simulink model "FOC_Motor_Sensorless"  (R2025b)
settings: Solver=VariableStepAuto  StartTime=0.0  StopTime=8  RelTol=1e-3
undefined symbols (not defined in the file or in its folder): adc, dataRange, encoder, inverter, paramAdcAmperePerCount, paramAdcCalibrationSamples, paramAdcCountAtZeroAmpere, paramAdcEnablecalibration, paramCurrentControlSatVoltage, paramOverCurrentDuration, paramOverCurrentEnable, paramOverCurrentLimit, paramPwmCompareAtZeroVolt, paramPwmCompareMax, paramPwmComparePerVolt, paramVelocityControlSatCurrent, PI_params, pmsm, PU_System, pwm, sampleTime
libraries: fl_lib x12, nesl_utility x12, mcbeeMathTransformLib x5, mcbcontrolslib x5, ee_lib x4, slpidlib x2, simulink x2, mcbhdlpositiondecoderlib x2, mcbplantlib x1, autolibpmsmexterior x1, eeGeneralControl x1, SignalEditorBlockLib x1
(part 1 of 2)
settings Model: DataDictionary=FoCFpgaData.sldd  ExtModeTrigDuration=100  LastModifiedBy=Admin
settings SolverCC: ZeroCrossAlgorithm=Adaptive  AlgebraicLoopSolver=TrustRegion
settings DataIOCC: LimitDataPoints=on  SaveFormat=Structure  SaveOutput=off  InspectSignalLogs=on  SaveTime=off  ReturnWorkspaceOutputs=off
settings OptimizationCC: DefaultParameterBehavior=Inlined  UseDivisionForNetSlopeComputation=on  GainParamInheritBuiltInType=on  UseFloatMulNetSlope=on  DefaultUnderspecifiedDataType=single  UseSpecifiedMinMax=on  InlineInvariantSignals=on  ReuseModelBlockBuffer=off  PassReuseOutputArgsAs=Individual arguments  ZeroExternalMemoryAtStartup=off  ZeroInternalMemoryAtStartup=off  NoFixptDivByZeroProtection=on  EfficientFloat2IntCast=on  LifeSpan=1  MaxStackSize=64  OptimizationLevel=level1  OptimizationCustomize=off  EfficientTunableParamExpr=on
settings DebuggingCC: IgnoredZcDiagnostic=none  SolverPrmCheckMsg=warning  InheritedTsInSrcMsg=none  ParameterPrecisionLossMsg=none  UnconnectedInputMsg=warning  UnconnectedOutputMsg=warning  UnconnectedLineMsg=warning  AllowSymbolicDim=off  SubsystemReferenceDiagnosticForUnitTest=warning  SFUnexpectedBacktrackingDiag=warning  SFNoUnconditionalDefaultTransitionDiag=warning  SFExecutionAtInitializationDiag=none  ArithmeticOperatorsInVariantConditions=warning
settings HardwareCC: ProdBitPerPointer=32.0  ProdBitPerSizeT=32.0  ProdBitPerPtrDiffT=32.0  ProdLargestAtomicInteger=Long  ProdWordSize=32.0  ProdLongLongMode=on  ProdHWDeviceType=ARM Compatible->ARM 10  TargetBitPerPointer=64.0  TargetBitPerSizeT=64.0  TargetBitPerPtrDiffT=64.0  TargetLongLongMode=on  TargetIntDivRoundTo=Zero  TargetEndianess=LittleEndian  TargetWordSize=64.0  TargetHWDeviceType=MATLAB Host  ProdEqTarget=off
settings ModelReferenceCC: EnableRefExpFcnMdlSchedulingChecks=on  PropagateSignalLabelsOutOfModel=off
settings SFSimCC: SimUseLocalCustomCode=off  MATLABDynamicMemAlloc=off  CustomCodeUndefinedFunction=UseInterfaceOnly
settings RTWCC: SystemTargetFile=ert.tlc  TemplateMakefile=ert_default_tmf  GenerateReport=on  RTWUseLocalCustomCode=off  BuildConfiguration=Faster Runs  IncludeHyperlinkInReport=on  LaunchReport=on  CodeProfilingSaveOptions=AllData  DataTypeReplacement=CDataTypesFixedWidth  TargetLang=C++  GenerateTraceInfo=on  GenerateCodeMetricsReport=on  GPUComputeCapability=3.5  DLArmComputeVersion=19.05  Description=Embedded Coder
settings CodeAppCC: ForceParamTrailComments=on  GenerateComments=off  IgnoreCustomStorageClasses=off  SimulinkDataObjDesc=on  CustomSymbolStrGlobalVar=rt$N$M  CustomSymbolStrType=$N$M  CustomSymbolStrFcn=$N$M$F  CustomSymbolStrFcnArg=$I$N$M  CustomSymbolStrMacro=$N$M  InsertBlockDesc=on
settings ERTTargetCC: RootIOFormat=Structure reference  ERTCustomFileTemplate=example_file_process.tlc  ERTFilePackagingFormat=CompactWithDataFile  PreserveExternInFcnDecls=off  EnableSignedLeftShifts=off  EnableSignedRightShifts=off  MaxIdInt64=INT64_MAX  MinIdInt64=INT64_MIN  MaxIdUint64=UINT64_MAX  MaxIdInt32=INT32_MAX  MinIdInt32=INT32_MIN  MaxIdUint32=UINT32_MAX  MaxIdInt16=INT16_MAX  MinIdInt16=INT16_MIN  MaxIdUint16=UINT16_MAX  MaxIdInt8=INT8_MAX  MinIdInt8=INT8_MIN  MaxIdUint8=UINT8_MAX  TargetLangStandard=C++17 (ISO)  MultiwordLength=2048.0  GenerateSampleERTMain=on  IncludeMdlTerminateFcn=off  CombineSignalStateStructs=on  CodeInterfacePackaging=C++ class  SubcomponentCodeInterfacePackaging=C++ class  SupportComplex=off  SupportNonInlinedSFcns=on
settings ConfigComp: CovMetricSettings=dw  CovSaveCumulativeToWorkspaceVar=on  CovSaveSingleToWorkspaceVar=on  CovExternalEMLEnable=off  CovSFcnEnable=off  PLC_TargetIDE=codesys35  PLC_MultiTBSigbuilderTimeRange=off  PLC_FoldFBCallOutputVar=off  PLC_RemoveUnusedSSMethodCallArguments=off  PLC_UseCallOutputArgSyntax=off  PLC_EnableUnsignedAndDoubleTypes=off  PLC_EnableUDTSplitting=off  PLC_MaxFieldsInUDT=500.0  PLC_InlineEnumCastFunction=off  PLC_RTWMaxIdLength=31.0  PLC_RollThreshold=5.0  PLC_ActiveTab=0.0  PLC_EnableStringLiteralTB=on  PLC_Enable64bitIntSupport=off
settings SimscapeCC: SimscapeNormalizeSystem=off  SimscapeNominalValues="[{\"value\":\"10\",\"unit\":\"V\"},{\"value\":\"1\",\"unit\":\"A\"},{\"value\":\"10\",\"unit\":\"N*m\"},{\"value\":\"10\",\"unit\":\"bar\"},{\"value\":\"100\",\"unit\":\"kJ/kg\"},{\"value\":\"1\",\"unit\":\"kW\"},{\"value\":\"300\",\"unit\":\"K\"},{\"value\":\"100\",\"unit\":\"cm^3/s\"},{\"value\":\"1\",\"unit\":\"kN\"},{\"value\":\"1\",\"unit\":\"g/cm^3\"},{\"value\":\"1\",\"unit\":\"l\"},{\"value\":\"1\",\"unit\":\"cm^2\"},{\"value\":\"60\",\"unit\":\"Hz\"}]"
settings SettingsController: CoderTargetData=[]

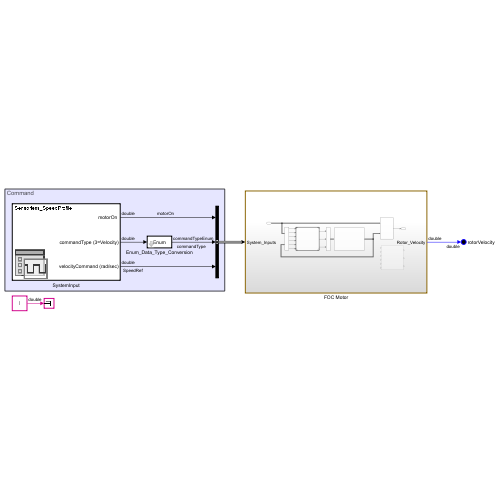
[thumbnail: Simulink's stored preview of the top-level diagram]
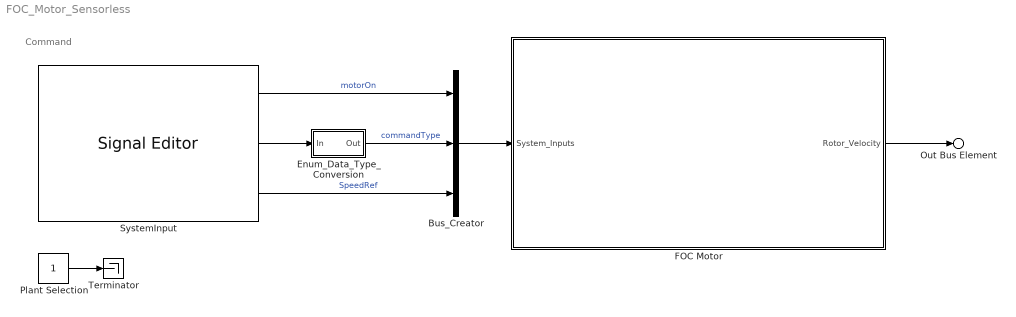
== system FOC_Motor_Sensorless ==
  note: Command
  Bus_Creator : BusCreator  Inputs=3
  Enum_Data_Type_Conversion : Subsystem  mask(Convert to enumerated data type){dataTypeStr=Enum: commandTypeEnum}
      mask prompts: dataTypeStr "Output data type"
      mask Display: disp('Enum')
  FOC Motor : Subsystem
  Plant Selection : Constant
  SystemInput : SignalEditorBlockLib/Signal Editor  FileName=SystemInputFO.mat  ActiveScenario=Sensorless_SpeedProfile  ActiveSignal=motorOn  IsBus=off  OutputBusObjectStr=Bus: BusObject  SampleTime=0  Interpolate=off  ZeroCross=off  OutputAfterFinalValue=Setting to zero  Unit=inherit  PreserveSignalName=on  ApplySigPropsToAllScenarios=off  ApplySigPropsToAllSignals=off  SignalPropertySource=Dialog parameters
  Terminator : Terminator
  Out Bus Element : Outport  PortName=rotorVelocity
  wires:
  Plant Selection/1 -> Terminator/1
  FOC Motor/1(Rotor_Velocity) -> Out Bus Element/1
  Bus_Creator/1 -> FOC Motor/1(System_Inputs)
  SystemInput/3 -> Bus_Creator/3  "SpeedRef"
  Enum_Data_Type_Conversion/1(Out) -> Bus_Creator/2  "commandType"
  SystemInput/2 -> Enum_Data_Type_Conversion/1(In)
  SystemInput/1 -> Bus_Creator/1  "motorOn"

== system FOC_Motor_Sensorless/Enum_Data_Type_Conversion ==
  note: Enum Data Type Conversion
  In : Inport
  Enum_Data_Type : DataTypeConversion  OutDataTypeStr=Enum: commandTypeEnum  SaturateOnIntegerOverflow=off  RndMeth=Floor
  Int32_Data_Type : DataTypeConversion  OutDataTypeStr=int32  SaturateOnIntegerOverflow=off  RndMeth=Floor
  Out : Outport
  wires:
  In/1 -> Int32_Data_Type/1
  Int32_Data_Type/1 -> Enum_Data_Type/1
  Enum_Data_Type/1 -> Out/1

== system FOC_Motor_Sensorless/FOC Motor ==
  note: Permanent Magnet Synchronous Motor Field Oriented Control
  System_Inputs : Inport
  Continuous_To_Discrete : Subsystem
      mask Display: fprintf('C/D')
  Controller_Algorithm_Local : Subsystem  Commented=on  TreatAsAtomicUnit=on  DataTypeOverrideAppliesTo=Fixed-point
      mask Display: image('MC_Mask.jpg');
  Discrete_To_Continuous : Subsystem  Description=""
      mask Display: fprintf('D/C')
  Model : ModelReference  ModelNameDialog=Controller_Algorithm_Local_FO.slx  SimulationMode=Normal  ModelReferenceVersion=1.4
  Motor_And_Load : Subsystem
      mask Display: image('mcb_pmsmfoc_motor.png');
  Verify_Outputs : Subsystem  Description=|
      | System Analysis for Speed Control Design
      | 
      | Analyize and plot signals used to analyize performance of
      | speed  control designs
      mask Display: fprintf('Verify\nOutputs')
  Rotor_Velocity : Outport
  wires:
  Continuous_To_Discrete/5(Encoder_Index_Found) -> Model/5
  Continuous_To_Discrete/4(ADC_Count) -> Model/4
  Motor_And_Load/1(Out) -> Continuous_To_Discrete/2(Motor_Measurements), Verify_Outputs/2(System_Measurements)
  Model/1 -> Discrete_To_Continuous/1(Controller_Mode)
  Discrete_To_Continuous/1(Motor_Commands) -> Motor_And_Load/1(Controller)
  Model/3 -> Discrete_To_Continuous/3(PWM_Compare)
  Continuous_To_Discrete/1(Motor_On) -> Model/1
  System_Inputs/1 -> Continuous_To_Discrete/1(System_Inputs), Verify_Outputs/1(System_Inputs)
  Continuous_To_Discrete/3(Velocity_Command) -> Model/3
  Verify_Outputs/1(Rotor_Velocity) -> Rotor_Velocity/1
  Continuous_To_Discrete/2(Command_Type) -> Model/2
  Continuous_To_Discrete/6(Encoder_Count) -> Model/6
  Model/2 -> Discrete_To_Continuous/2(Inverter_Enable)

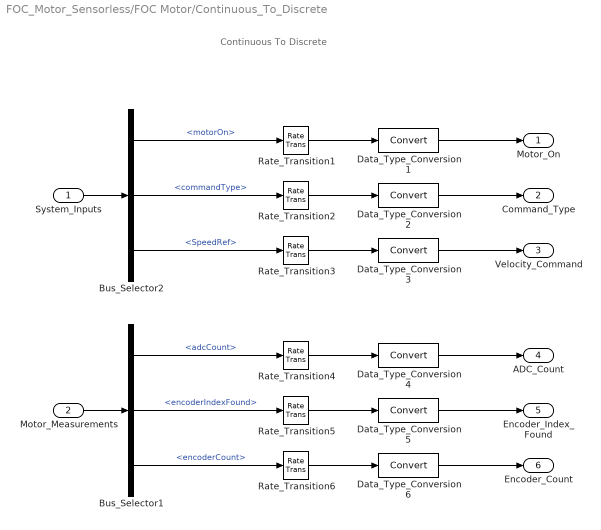
== system FOC_Motor_Sensorless/FOC Motor/Continuous_To_Discrete ==
  note: Continuous To Discrete
  System_Inputs : Inport
  Motor_Measurements : Inport  Port=2
  Bus_Selector1 : BusSelector  OutputSignals=adcCount,encoderIndexFound,encoderCount
  Bus_Selector2 : BusSelector  OutputSignals=motorOn,commandType,SpeedRef
  Data_Type_Conversion{1..6} (6 alike) : DataTypeConversion  SaturateOnIntegerOverflow=off  RndMeth=Floor
  Rate_Transition1 : RateTransition  Integrity=off  Deterministic=off
  Rate_Transition2 : RateTransition  Integrity=off  Deterministic=off
  Rate_Transition3 : RateTransition  Integrity=off  Deterministic=off
  Rate_Transition4 : RateTransition  Deterministic=off
  Rate_Transition5 : RateTransition  Deterministic=off
  Rate_Transition6 : RateTransition  Deterministic=off
  Motor_On : Outport
  Command_Type : Outport  Port=2
  Velocity_Command : Outport  Port=3
  ADC_Count : Outport  Port=4
  Encoder_Index_Found : Outport  Port=5
  Encoder_Count : Outport  Port=6
  wires:
  Bus_Selector2/3 -> Rate_Transition3/1  "<SpeedRef>"
  Bus_Selector2/2 -> Rate_Transition2/1  "<commandType>"
  Bus_Selector2/1 -> Rate_Transition1/1  "<motorOn>"
  System_Inputs/1 -> Bus_Selector2/1
  Bus_Selector1/3 -> Rate_Transition6/1  "<encoderCount>"
  Bus_Selector1/2 -> Rate_Transition5/1  "<encoderIndexFound>"
  Bus_Selector1/1 -> Rate_Transition4/1  "<adcCount>"
  Data_Type_Conversion6/1 -> Encoder_Count/1
  Data_Type_Conversion5/1 -> Encoder_Index_Found/1
  Rate_Transition6/1 -> Data_Type_Conversion6/1
  Rate_Transition5/1 -> Data_Type_Conversion5/1
  Rate_Transition1/1 -> Data_Type_Conversion1/1
  Data_Type_Conversion1/1 -> Motor_On/1
  Motor_Measurements/1 -> Bus_Selector1/1
  Data_Type_Conversion4/1 -> ADC_Count/1
  Rate_Transition4/1 -> Data_Type_Conversion4/1
  Rate_Transition3/1 -> Data_Type_Conversion3/1
  Data_Type_Conversion3/1 -> Velocity_Command/1
  Data_Type_Conversion2/1 -> Command_Type/1
  Rate_Transition2/1 -> Data_Type_Conversion2/1

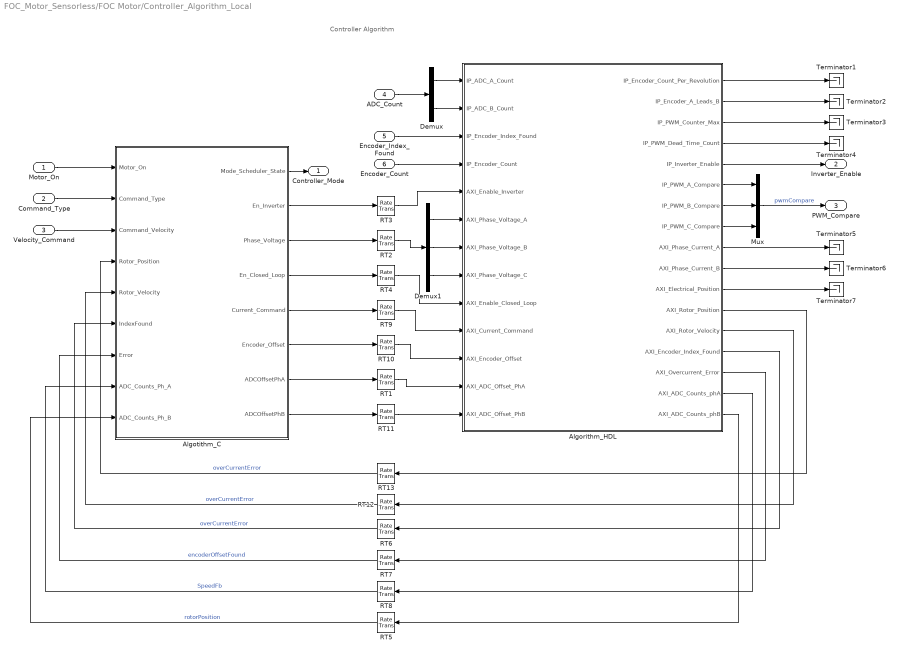
== system FOC_Motor_Sensorless/FOC Motor/Controller_Algorithm_Local ==
  note: Controller Algorithm
  Motor_On : Inport  SampleTime=sampleTime.VelocityControl  Interpolate=off
  Command_Type : Inport  Port=2  Interpolate=off
  Velocity_Command : Inport  Port=3
  ADC_Count : Inport  Port=4  PortDimensions=2  SampleTime=sampleTime.CurrentControl  Interpolate=off
  Encoder_Index_Found : Inport  Port=5  Interpolate=off
  Encoder_Count : Inport  Port=6  Interpolate=off
  Algorithm_HDL : Subsystem
  Algotithm_C : Subsystem
  Demux : Demux  Outputs=2
  Demux1 : Demux  Outputs=3
  Mux : Mux  Inputs=3
  RT{1..13} (13 alike) : RateTransition  Integrity=off
  Terminator{1..7} (7 alike) : Terminator
  Controller_Mode : Outport
  Inverter_Enable : Outport  Port=2
  PWM_Compare : Outport  Port=3
  wires:
  ADC_Count/1 -> Demux/1
  Mux/1 -> PWM_Compare/1  "pwmCompare"
  RT2/1 -> Demux1/1
  Motor_On/1 -> Algotithm_C/1(Motor_On)
  Command_Type/1 -> Algotithm_C/2(Command_Type)
  Velocity_Command/1 -> Algotithm_C/3(Command_Velocity)
  RT13/1 -> Algotithm_C/4(Rotor_Position)  "overCurrentError"
  RT12/1 -> Algotithm_C/5(Rotor_Velocity)  "overCurrentError"
  RT6/1 -> Algotithm_C/6(IndexFound)  "overCurrentError"
  RT7/1 -> Algotithm_C/7(Error)  "encoderOffsetFound"
  RT8/1 -> Algotithm_C/8(ADC_Counts_Ph_A)  "SpeedFb"
  RT5/1 -> Algotithm_C/9(ADC_Counts_Ph_B)  "rotorPosition"
  Algotithm_C/1(Mode_Scheduler_State) -> Controller_Mode/1
  Algotithm_C/2(En_Inverter) -> RT3/1
  Algotithm_C/3(Phase_Voltage) -> RT2/1
  Algotithm_C/4(En_Closed_Loop) -> RT4/1
  Algotithm_C/5(Current_Command) -> RT9/1
  Algotithm_C/6(Encoder_Offset) -> RT10/1
  Algotithm_C/7(ADCOffsetPhA) -> RT1/1
  Algotithm_C/8(ADCOffsetPhB) -> RT11/1
  Demux/1 -> Algorithm_HDL/1(IP_ADC_A_Count)
  Demux/2 -> Algorithm_HDL/2(IP_ADC_B_Count)
  Encoder_Index_Found/1 -> Algorithm_HDL/3(IP_Encoder_Index_Found)
  Encoder_Count/1 -> Algorithm_HDL/4(IP_Encoder_Count)
  RT3/1 -> Algorithm_HDL/5(AXI_Enable_Inverter)
  Demux1/1 -> Algorithm_HDL/6(AXI_Phase_Voltage_A)
  Demux1/2 -> Algorithm_HDL/7(AXI_Phase_Voltage_B)
  Demux1/3 -> Algorithm_HDL/8(AXI_Phase_Voltage_C)
  RT4/1 -> Algorithm_HDL/9(AXI_Enable_Closed_Loop)
  RT9/1 -> Algorithm_HDL/10(AXI_Current_Command)
  RT10/1 -> Algorithm_HDL/11(AXI_Encoder_Offset)
  RT1/1 -> Algorithm_HDL/12(AXI_ADC_Offset_PhA)
  RT11/1 -> Algorithm_HDL/13(AXI_ADC_Offset_PhB)
  Algorithm_HDL/1(IP_Encoder_Count_Per_Revolution) -> Terminator1/1
  Algorithm_HDL/2(IP_Encoder_A_Leads_B) -> Terminator2/1
  Algorithm_HDL/3(IP_PWM_Counter_Max) -> Terminator3/1
  Algorithm_HDL/4(IP_PWM_Dead_Time_Count) -> Terminator4/1
  Algorithm_HDL/5(IP_Inverter_Enable) -> Inverter_Enable/1
  Algorithm_HDL/6(IP_PWM_A_Compare) -> Mux/1
  Algorithm_HDL/7(IP_PWM_B_Compare) -> Mux/2
  Algorithm_HDL/8(IP_PWM_C_Compare) -> Mux/3
  Algorithm_HDL/9(AXI_Phase_Current_A) -> Terminator5/1
  Algorithm_HDL/10(AXI_Phase_Current_B) -> Terminator6/1
  Algorithm_HDL/11(AXI_Electrical_Position) -> Terminator7/1
  Algorithm_HDL/12(AXI_Rotor_Position) -> RT13/1
  Algorithm_HDL/13(AXI_Rotor_Velocity) -> RT12/1
  Algorithm_HDL/14(AXI_Encoder_Index_Found) -> RT6/1
  Algorithm_HDL/15(AXI_Overcurrent_Error) -> RT7/1
  Algorithm_HDL/16(AXI_ADC_Counts_phA) -> RT8/1
  Algorithm_HDL/17(AXI_ADC_Counts_phB) -> RT5/1

== system FOC_Motor_Sensorless/FOC Motor/Discrete_To_Continuous ==
  note: Discrete To Continuous
  Controller_Mode : Inport
  Inverter_Enable : Inport  Port=2
  PWM_Compare : Inport  Port=3
  Bus_Creator1 : BusCreator  Inputs=3
  Data_Type_Conversion1 : DataTypeConversion  OutDataTypeStr=Enum: modeSchedulerEnum  SaturateOnIntegerOverflow=off  RndMeth=Floor
  Data_Type_Conversion2 : DataTypeConversion  SaturateOnIntegerOverflow=off  RndMeth=Floor
  Data_Type_Conversion3 : DataTypeConversion  SaturateOnIntegerOverflow=off  RndMeth=Floor
  Rate_Transition1 : RateTransition  Integrity=off  Deterministic=off
  Rate_Transition2 : RateTransition  Deterministic=off
  Rate_Transition3 : RateTransition  Deterministic=off
  Motor_Commands : Outport
  wires:
  Controller_Mode/1 -> Data_Type_Conversion1/1
  Data_Type_Conversion1/1 -> Rate_Transition1/1
  Rate_Transition3/1 -> Bus_Creator1/3  "pwmCompare"
  Rate_Transition2/1 -> Bus_Creator1/2  "inverterEnable"
  PWM_Compare/1 -> Data_Type_Conversion3/1
  Data_Type_Conversion3/1 -> Rate_Transition3/1
  Inverter_Enable/1 -> Data_Type_Conversion2/1
  Data_Type_Conversion2/1 -> Rate_Transition2/1
  Bus_Creator1/1 -> Motor_Commands/1
  Rate_Transition1/1 -> Bus_Creator1/1  "controllerMode"

== system FOC_Motor_Sensorless/FOC Motor/Motor_And_Load ==
  note: Inverter Motor and Load
  Controller : Inport
  Bus_Creator2 : BusCreator  Inputs=6
  Bus_Selector4 : BusSelector  OutputSignals=pwmCompare,inverterEnable
  Data Type Conversion : DataTypeConversion  OutDataTypeStr=boolean  SaturateOnIntegerOverflow=off  RndMeth=Floor
  Demux : Demux  Outputs=3
  Load_Profile (Torque) : Subsystem
  "Plant " : Subsystem  Variant=on
      mask Display: image('FOC_Motor_Mask.jpg');
  RT1 : RateTransition  Deterministic=off  OutPortSampleTime=sampleTime.CurrentControl/2
  RT2 : RateTransition  Deterministic=off  OutPortSampleTime=sampleTime.CurrentControl/2
  RT3 : RateTransition  Deterministic=off  OutPortSampleTime=sampleTime.CurrentControl/2
  Radio Button : RadioButtonGroup  SelectedLabel=MCB  ButtonGroupName=Inverter+Motor Plant Model
  Rate Transition : RateTransition  Deterministic=off  OutPortSampleTime=sampleTime.CurrentControl/2
  Rate Transition1 : RateTransition  Deterministic=off  OutPortSampleTime=sampleTime.CurrentControl/2
  Rate Transition2 : RateTransition  Deterministic=off  OutPortSampleTime=sampleTime.CurrentControl/2
  Sensor_Measurements : Subsystem
      mask Display: image('Sensor_Mask.jpg');
  Out : Outport
  wires:
  Bus_Creator2/1 -> Out/1
  Controller/1 -> Bus_Selector4/1, Bus_Creator2/1  "controller"
  Bus_Selector4/1 -> Rate Transition/1  "<pwmCompare>"
  Sensor_Measurements/1(Sim_fb) -> Demux/1
  Demux/1 -> Bus_Creator2/2  "adcCount"
  Demux/3 -> Data Type Conversion/1
  Data Type Conversion/1 -> Bus_Creator2/4  "encoderIndexFound"
  Demux/2 -> Bus_Creator2/3  "encoderCount"
  "Plant "/1(Theta) -> RT3/1
  RT3/1 -> Sensor_Measurements/1(Info)
  Rate Transition/1 -> "Plant "/1(Vabc)
  "Plant "/2(Iabc) -> RT1/1  "Iabc"
  Rate Transition1/1 -> "Plant "/3(Load)
  Load_Profile (Torque)/1(Load_Trq) -> Rate Transition1/1
  RT1/1 -> Bus_Creator2/5, Sensor_Measurements/2(PhaseCurr)  "phasecurrents"
  RT2/1 -> Bus_Creator2/6  "motorspeed"
  "Plant "/3(MotorSpeed) -> RT2/1  "motorspeed"
  Bus_Selector4/2 -> Rate Transition2/1  "<inverterEnable>"
  Rate Transition2/1 -> "Plant "/2(InverterEnable)

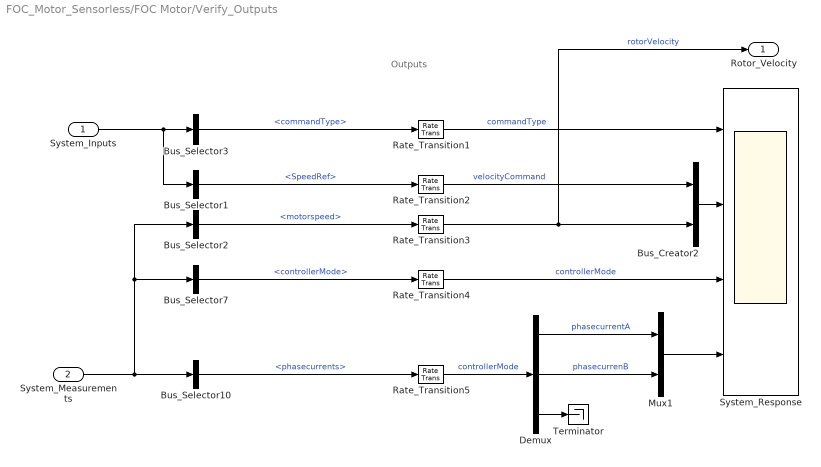
== system FOC_Motor_Sensorless/FOC Motor/Verify_Outputs ==
  note: Outputs
  System_Inputs : Inport
  System_Measurements : Inport  Port=2
  Bus_Creator2 : BusCreator  Inputs=2
  Bus_Selector1 : BusSelector  OutputSignals=SpeedRef
  Bus_Selector10 : BusSelector  OutputSignals=phasecurrents
  Bus_Selector2 : BusSelector  OutputSignals=motorspeed
  Bus_Selector3 : BusSelector  OutputSignals=commandType
  Bus_Selector7 : BusSelector  OutputSignals=controller.controllerMode
  Demux : Demux  Outputs=3
  Mux1 : Mux  Inputs=2
  Rate_Transition{1..5} (5 alike) : RateTransition  Integrity=off
  System_Response : Scope  NumInputPorts=4
      settings: SampleTime=1e-3  TimeUnits=Metric (based on Time Span)  Title=Command Type  ActiveDisplayYMinimum=2  ActiveDisplayYMaximum=4
      settings: AttributesFormatString=|
      | --------------------------------------
      | SampleTime = %<SampleTime>
  Terminator : Terminator
  Rotor_Velocity : Outport
  wires:
  Bus_Selector3/1 -> Rate_Transition1/1  "<commandType>"
  Bus_Selector7/1 -> Rate_Transition4/1  "<controllerMode>"
  Bus_Selector1/1 -> Rate_Transition2/1  "<SpeedRef>"
  Mux1/1 -> System_Response/4
  Rate_Transition4/1 -> System_Response/3  "controllerMode"
  Bus_Creator2/1 -> System_Response/2
  Rate_Transition1/1 -> System_Response/1  "commandType"
  System_Inputs/1 -> Bus_Selector1/1, Bus_Selector3/1
  System_Measurements/1 -> Bus_Selector2/1, Bus_Selector7/1, Bus_Selector10/1
  Rate_Transition2/1 -> Bus_Creator2/1  "velocityCommand"
  Rate_Transition3/1 -> Rotor_Velocity/1, Bus_Creator2/2  "rotorVelocity"
  Demux/1 -> Mux1/1  "phasecurrentA"
  Demux/2 -> Mux1/2  "phasecurrenB"
  Bus_Selector2/1 -> Rate_Transition3/1  "<motorspeed>"
  Bus_Selector10/1 -> Rate_Transition5/1  "<phasecurrents>"
  Rate_Transition5/1 -> Demux/1  "controllerMode"
  Demux/3 -> Terminator/1

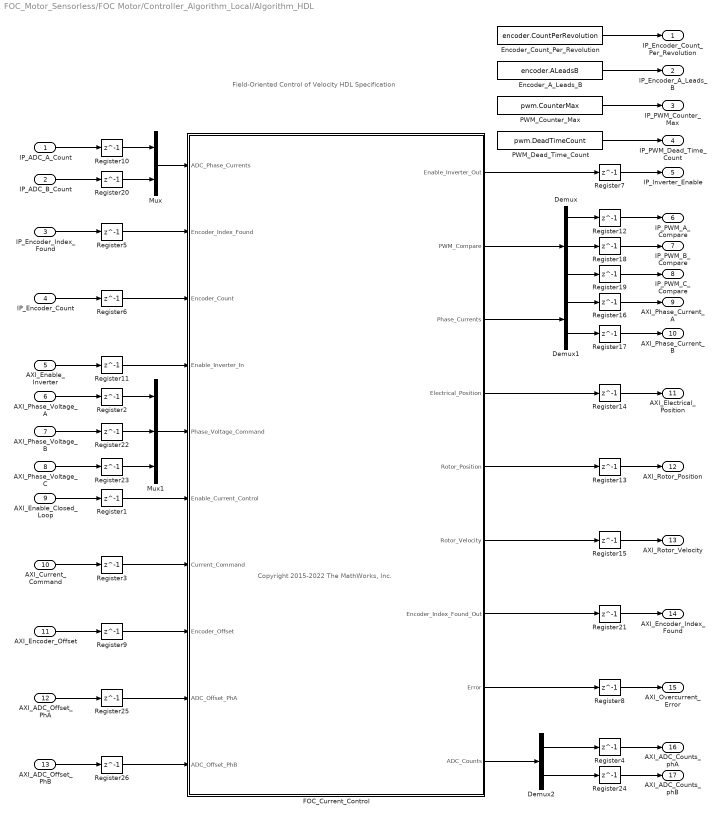
== system FOC_Motor_Sensorless/FOC Motor/Controller_Algorithm_Local/Algorithm_HDL ==
  note: Copyright 2015-2022 The MathWorks, Inc.
  note: Field-Oriented Control of Velocity
      | HDL Specification
  IP_ADC_A_Count : Inport  PortDimensions=1  Interpolate=off
  IP_ADC_B_Count : Inport  Port=2  PortDimensions=1  Interpolate=off
  IP_Encoder_Index_Found : Inport  Port=3  Interpolate=off
  IP_Encoder_Count : Inport  Port=4  Interpolate=off
  AXI_Enable_Inverter : Inport  Port=5
  AXI_Phase_Voltage_A : Inport  Port=6
  AXI_Phase_Voltage_B : Inport  Port=7
  AXI_Phase_Voltage_C : Inport  Port=8
  AXI_Enable_Closed_Loop : Inport  Port=9
  AXI_Current_Command : Inport  Port=10
  AXI_Encoder_Offset : Inport  Port=11
  AXI_ADC_Offset_PhA : Inport  Port=12
  AXI_ADC_Offset_PhB : Inport  Port=13
  Demux : Demux  Outputs=3
  Demux1 : Demux  Outputs=2
  Demux2 : Demux  Outputs=2
  Encoder_A_Leads_B : Constant  Value=encoder.ALeadsB  OutDataTypeStr=fixdt(0,1,0)  SampleTime=-1
  Encoder_Count_Per_Revolution : Constant  Value=encoder.CountPerRevolution  OutDataTypeStr=fixdt(0,15,0)  SampleTime=-1
  FOC_Current_Control : Subsystem
  Mux : Mux  Inputs=2
  Mux1 : Mux  Inputs=3
  PWM_Counter_Max : Constant  Value=pwm.CounterMax  OutDataTypeStr=uint16  SampleTime=-1
  PWM_Dead_Time_Count : Constant  Value=pwm.DeadTimeCount  OutDataTypeStr=uint8  SampleTime=-1
  Register{1..26} (26 alike) : Delay  DelayLength=1
  IP_Encoder_Count_Per_Revolution : Outport  VectorParamsAs1DForOutWhenUnconnected=off
  IP_Encoder_A_Leads_B : Outport  Port=2  VectorParamsAs1DForOutWhenUnconnected=off
  IP_PWM_Counter_Max : Outport  Port=3  VectorParamsAs1DForOutWhenUnconnected=off
  IP_PWM_Dead_Time_Count : Outport  Port=4  VectorParamsAs1DForOutWhenUnconnected=off
  IP_Inverter_Enable : Outport  Port=5  VectorParamsAs1DForOutWhenUnconnected=off
  IP_PWM_A_Compare : Outport  Port=6  VectorParamsAs1DForOutWhenUnconnected=off
  IP_PWM_B_Compare : Outport  Port=7  VectorParamsAs1DForOutWhenUnconnected=off
  IP_PWM_C_Compare : Outport  Port=8  VectorParamsAs1DForOutWhenUnconnected=off
  AXI_Phase_Current_A : Outport  Port=9  VectorParamsAs1DForOutWhenUnconnected=off
  AXI_Phase_Current_B : Outport  Port=10  VectorParamsAs1DForOutWhenUnconnected=off
  AXI_Electrical_Position : Outport  Port=11  VectorParamsAs1DForOutWhenUnconnected=off
  AXI_Rotor_Position : Outport  Port=12  VectorParamsAs1DForOutWhenUnconnected=off
  AXI_Rotor_Velocity : Outport  Port=13  VectorParamsAs1DForOutWhenUnconnected=off
  AXI_Encoder_Index_Found : Outport  Port=14  VectorParamsAs1DForOutWhenUnconnected=off
  AXI_Overcurrent_Error : Outport  Port=15  VectorParamsAs1DForOutWhenUnconnected=off
  AXI_ADC_Counts_phA : Outport  Port=16  VectorParamsAs1DForOutWhenUnconnected=off
  AXI_ADC_Counts_phB : Outport  Port=17  VectorParamsAs1DForOutWhenUnconnected=off
  wires:
  Mux/1 -> FOC_Current_Control/1(ADC_Phase_Currents)
  Register21/1 -> AXI_Encoder_Index_Found/1
  Encoder_Count_Per_Revolution/1 -> IP_Encoder_Count_Per_Revolution/1
  Register13/1 -> AXI_Rotor_Position/1
  IP_Encoder_Count/1 -> Register6/1
  Demux/2 -> Register18/1
  FOC_Current_Control/6(Rotor_Velocity) -> Register15/1
  Demux2/1 -> Register4/1
  Register22/1 -> Mux1/2
  FOC_Current_Control/7(Encoder_Index_Found_Out) -> Register21/1
  FOC_Current_Control/2(PWM_Compare) -> Demux/1
  FOC_Current_Control/4(Electrical_Position) -> Register14/1
  Register3/1 -> FOC_Current_Control/7(Current_Command)
  FOC_Current_Control/1(Enable_Inverter_Out) -> Register7/1
  Register10/1 -> Mux/1
  AXI_ADC_Offset_PhA/1 -> Register25/1
  Demux/1 -> Register12/1
  Register6/1 -> FOC_Current_Control/3(Encoder_Count)
  IP_ADC_B_Count/1 -> Register20/1
  Register14/1 -> AXI_Electrical_Position/1
  Register9/1 -> FOC_Current_Control/8(Encoder_Offset)
  Register11/1 -> FOC_Current_Control/4(Enable_Inverter_In)
  FOC_Current_Control/3(Phase_Currents) -> Demux1/1
  Demux1/1 -> Register16/1
  Encoder_A_Leads_B/1 -> IP_Encoder_A_Leads_B/1
  Demux1/2 -> Register17/1
  Register23/1 -> Mux1/3
  AXI_Phase_Voltage_B/1 -> Register22/1
  FOC_Current_Control/5(Rotor_Position) -> Register13/1
  Register26/1 -> FOC_Current_Control/10(ADC_Offset_PhB)
  AXI_ADC_Offset_PhB/1 -> Register26/1
  Register15/1 -> AXI_Rotor_Velocity/1
  AXI_Phase_Voltage_A/1 -> Register2/1
  IP_ADC_A_Count/1 -> Register10/1
  Register19/1 -> IP_PWM_C_Compare/1
  Register24/1 -> AXI_ADC_Counts_phB/1
  PWM_Counter_Max/1 -> IP_PWM_Counter_Max/1
  Register16/1 -> AXI_Phase_Current_A/1
  AXI_Phase_Voltage_C/1 -> Register23/1
  Register18/1 -> IP_PWM_B_Compare/1
  Register25/1 -> FOC_Current_Control/9(ADC_Offset_PhA)
  Demux2/2 -> Register24/1
  Register20/1 -> Mux/2
  PWM_Dead_Time_Count/1 -> IP_PWM_Dead_Time_Count/1
  FOC_Current_Control/8(Error) -> Register8/1
  Register8/1 -> AXI_Overcurrent_Error/1
  Register5/1 -> FOC_Current_Control/2(Encoder_Index_Found)
  Mux1/1 -> FOC_Current_Control/5(Phase_Voltage_Command)
  Register4/1 -> AXI_ADC_Counts_phA/1
  FOC_Current_Control/9(ADC_Counts) -> Demux2/1
  AXI_Enable_Closed_Loop/1 -> Register1/1
  Demux/3 -> Register19/1
  AXI_Current_Command/1 -> Register3/1
  IP_Encoder_Index_Found/1 -> Register5/1
  Register17/1 -> AXI_Phase_Current_B/1
  AXI_Encoder_Offset/1 -> Register9/1
  AXI_Enable_Inverter/1 -> Register11/1
  Register1/1 -> FOC_Current_Control/6(Enable_Current_Control)
  Register2/1 -> Mux1/1
  Register7/1 -> IP_Inverter_Enable/1
  Register12/1 -> IP_PWM_A_Compare/1

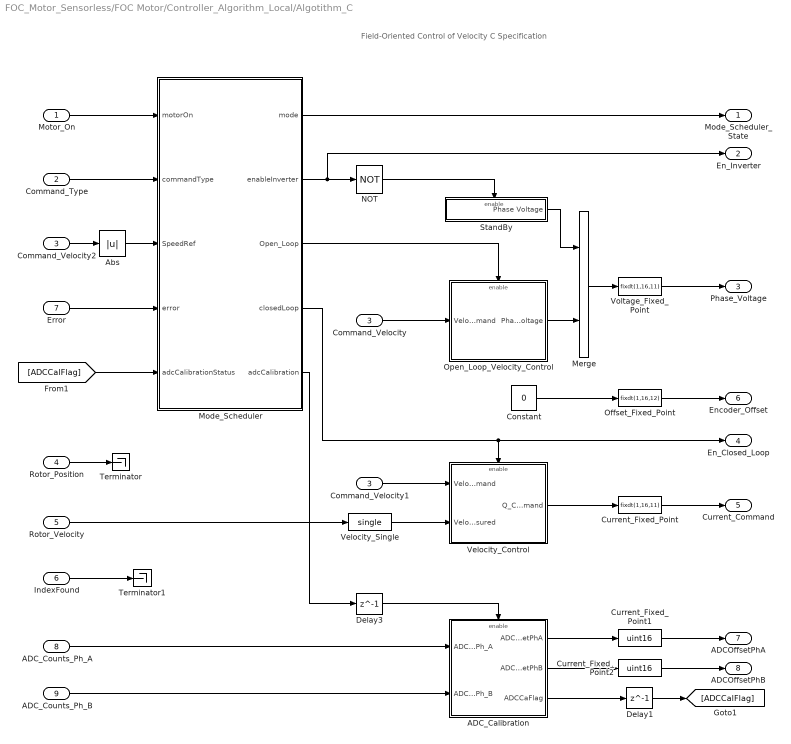
== system FOC_Motor_Sensorless/FOC Motor/Controller_Algorithm_Local/Algotithm_C ==
  note: Field-Oriented Control of Velocity
      | C Specification
  Motor_On : Inport  OutDataTypeStr=boolean
  Command_Type : Inport  Port=2  OutDataTypeStr=Enum: commandTypeEnum
  Command_Velocity : Inport  Port=3
  Rotor_Position : Inport  Port=4  OutMin=0  OutMax=2*pi  OutDataTypeStr=fixdt(1,16,12)  SampleTime=sampleTime.VelocityControl
  Rotor_Velocity : Inport  Port=5  OutMin=dataRange.RotorVelocity.Min  OutMax=dataRange.RotorVelocity.Max  OutDataTypeStr=fixdt(1,16,5)
  IndexFound : Inport  Port=6  OutDataTypeStr=boolean
  Error : Inport  Port=7  OutDataTypeStr=boolean
  ADC_Counts_Ph_A : Inport  Port=8  OutDataTypeStr=uint16
  ADC_Counts_Ph_B : Inport  Port=9  OutDataTypeStr=uint16
  ADC_Calibration : Subsystem
      mask Display: fprintf('ADC\nCalibration')
  Abs : Abs  SaturateOnIntegerOverflow=off
  Command_Velocity1 : InportShadow  Port=3
  Command_Velocity2 : InportShadow  Port=3
  Constant : Constant  Value=0  OutDataTypeStr=single  SampleTime=-1
  Current_Fixed_Point : DataTypeConversion  OutMin=dataRange.PhaseCurrent.Min  OutMax=dataRange.PhaseCurrent.Max  OutDataTypeStr=fixdt(1,16,11)  SaturateOnIntegerOverflow=off  RndMeth=Floor
  Current_Fixed_Point1 : DataTypeConversion  OutDataTypeStr=uint16  SaturateOnIntegerOverflow=off  RndMeth=Floor
  Current_Fixed_Point2 : DataTypeConversion  OutDataTypeStr=uint16  SaturateOnIntegerOverflow=off  RndMeth=Floor
  Delay1 : Delay  DelayLength=1
  Delay3 : Delay  DelayLength=1
  Merge : Merge
      mask Display: disp(' ')
  Mode_Scheduler : Stateflow chart  TreatAsAtomicUnit=on
  NOT : Logic  Operator=NOT  IconShape=distinctive  AllPortsSameDT=off  OutDataTypeStr=boolean
  Offset_Fixed_Point : DataTypeConversion  OutMin=0  OutMax=2*pi  OutDataTypeStr=fixdt(1,16,12)  SaturateOnIntegerOverflow=off  RndMeth=Floor
  Open_Loop_Velocity_Control : Subsystem  TreatAsAtomicUnit=on
      settings: RTWFcnNameOpts=User specified  FunctionInterfaceSpec=Allow arguments (Optimized)
      mask Display: fprintf('Open Loop\nVelocity\nControl')
  StandBy : Subsystem  Description=Stand By mode for controller outputs constant phase voltages.  TreatAsAtomicUnit=on
      mask Display: fprintf('Disabled')
  Terminator : Terminator
  Terminator1 : Terminator
  Velocity_Control : Subsystem
      mask Display: fprintf('Velocity\nControl')
  Velocity_Single : DataTypeConversion  OutDataTypeStr=single  SaturateOnIntegerOverflow=off  RndMeth=Floor
  Voltage_Fixed_Point : DataTypeConversion  OutMin=dataRange.DqVoltage.Min  OutMax=dataRange.DqVoltage.Max  OutDataTypeStr=fixdt(1,16,11)  SaturateOnIntegerOverflow=off  RndMeth=Floor
  Mode_Scheduler_State : Outport  VectorParamsAs1DForOutWhenUnconnected=off
  En_Inverter : Outport  Port=2  VectorParamsAs1DForOutWhenUnconnected=off
  Phase_Voltage : Outport  Port=3  VectorParamsAs1DForOutWhenUnconnected=off
  En_Closed_Loop : Outport  Port=4  VectorParamsAs1DForOutWhenUnconnected=off
  Current_Command : Outport  Port=5  VectorParamsAs1DForOutWhenUnconnected=off
  Encoder_Offset : Outport  Port=6  VectorParamsAs1DForOutWhenUnconnected=off
  ADCOffsetPhA : Outport  Port=7  InitialOutput=0  VectorParamsAs1DForOutWhenUnconnected=off
  ADCOffsetPhB : Outport  Port=8  InitialOutput=0  VectorParamsAs1DForOutWhenUnconnected=off
  wires:
  StandBy/1(Phase Voltage) -> Merge/1
  ADC_Counts_Ph_A/1 -> ADC_Calibration/1(ADC_Counts_Ph_A)
  Mode_Scheduler/1(mode) -> Mode_Scheduler_State/1
  Abs/1 -> Mode_Scheduler/3(SpeedRef)
  Mode_Scheduler/4(" closedLoop") -> Velocity_Control/Enable, En_Closed_Loop/1
  ADC_Counts_Ph_B/1 -> ADC_Calibration/2(ADC_Counts_Ph_B)
  Command_Velocity/1 -> Open_Loop_Velocity_Control/1(Velocity_Command)
  Motor_On/1 -> Mode_Scheduler/1(motorOn)
  Rotor_Position/1 -> Terminator/1
  Velocity_Control/1(Q_Current_Command) -> Current_Fixed_Point/1
  Mode_Scheduler/2(" enableInverter") -> En_Inverter/1, NOT/1
  Mode_Scheduler/5(adcCalibration) -> Delay3/1
  Mode_Scheduler/3(" Open_Loop") -> Open_Loop_Velocity_Control/Enable
  Current_Fixed_Point/1 -> Current_Command/1
  ADC_Calibration/2(ADCOffsetPhB) -> Current_Fixed_Point2/1
  Command_Velocity2/1 -> Abs/1
  Command_Type/1 -> Mode_Scheduler/2(commandType)
  Merge/1 -> Voltage_Fixed_Point/1
  Current_Fixed_Point1/1 -> ADCOffsetPhA/1
  Error/1 -> Mode_Scheduler/4(error)
  NOT/1 -> StandBy/Enable
  IndexFound/1 -> Terminator1/1
  Constant/1 -> Offset_Fixed_Point/1
  Rotor_Velocity/1 -> Velocity_Single/1
  Current_Fixed_Point2/1 -> ADCOffsetPhB/1
  Offset_Fixed_Point/1 -> Encoder_Offset/1
  [ADCCalFlag] -> Mode_Scheduler/5(adcCalibrationStatus)
  Voltage_Fixed_Point/1 -> Phase_Voltage/1
  Command_Velocity1/1 -> Velocity_Control/1(Velocity_Command)
  Delay3/1 -> ADC_Calibration/Enable
  Open_Loop_Velocity_Control/1(Phase_Voltage) -> Merge/2
  Delay1/1 -> [ADCCalFlag]
  ADC_Calibration/1(ADCOffsetPhA) -> Current_Fixed_Point1/1
  ADC_Calibration/3(ADCCaFlag) -> Delay1/1
  Velocity_Single/1 -> Velocity_Control/2(Velocity_Measured)

== system FOC_Motor_Sensorless/FOC Motor/Motor_And_Load/Load_Profile (Torque) ==
  Data Type Conversion : DataTypeConversion  OutDataTypeStr=single  SaturateOnIntegerOverflow=off  RndMeth=Floor
  IIR Filter : mcbcontrolslib/IIR Filter  VariantControl=Low Pass Filter  VariantSelect=Low-pass  FilterConstantInputType=Specify via dialog  Filter_constant=0.01  InitialOutput=Specify via dialog  InitialOutputValue=0  ExternalReset=none  advancedSettings=off  Ts=50e-6  cutOff_freq=32.1525
  No_load_during_Standby : Step  Time=(paramAdcCalibrationSamples+1)*sampleTime.VelocityControl  SampleTime=sampleTime.CurrentControl/2
  No_load_load_selctor : Step  Time=7  Before=1  After=0  SampleTime=sampleTime.CurrentControl/2
  Noload : Constant  Value=0  SampleTime=sampleTime.CurrentControl/2
  Noload1 : Constant  Value=0  SampleTime=sampleTime.CurrentControl/2
  Switch : Switch  Criteria=u2 > Threshold  SaturateOnIntegerOverflow=off  InputSameDT=off
  Switch1 : Switch  Criteria=u2 > Threshold  SaturateOnIntegerOverflow=off  InputSameDT=off
  T_load : Step  Time=4  Before=0.1*pmsm.T_rated  After=0.2*pmsm.T_rated  SampleTime=sampleTime.CurrentControl/2
  Load_Trq : Outport  VectorParamsAs1DForOutWhenUnconnected=off
  wires:
  Data Type Conversion/1 -> IIR Filter/1
  IIR Filter/1 -> Load_Trq/1
  T_load/1 -> Switch/1
  No_load_load_selctor/1 -> Switch/2
  Noload/1 -> Switch/3
  Switch1/1 -> Data Type Conversion/1
  Switch/1 -> Switch1/1
  Noload1/1 -> Switch1/3
  No_load_during_Standby/1 -> Switch1/2

== system FOC_Motor_Sensorless/FOC Motor/Motor_And_Load/Plant  ==
  Vabc : Inport
  InverterEnable : Inport  Port=2
  Load : Inport  Port=3
  MCB : Subsystem  VariantControl=(get_param(['FOC_Motor_Sensorless' '/Plant Selection'], 'Value') == '1')
  Simscape : Subsystem  VariantControl=(get_param(['FOC_Motor_Sensorless' '/Plant Selection'], 'Value') == '2')
  Theta : Outport
  Iabc : Outport  Port=2
  MotorSpeed : Outport  Port=3

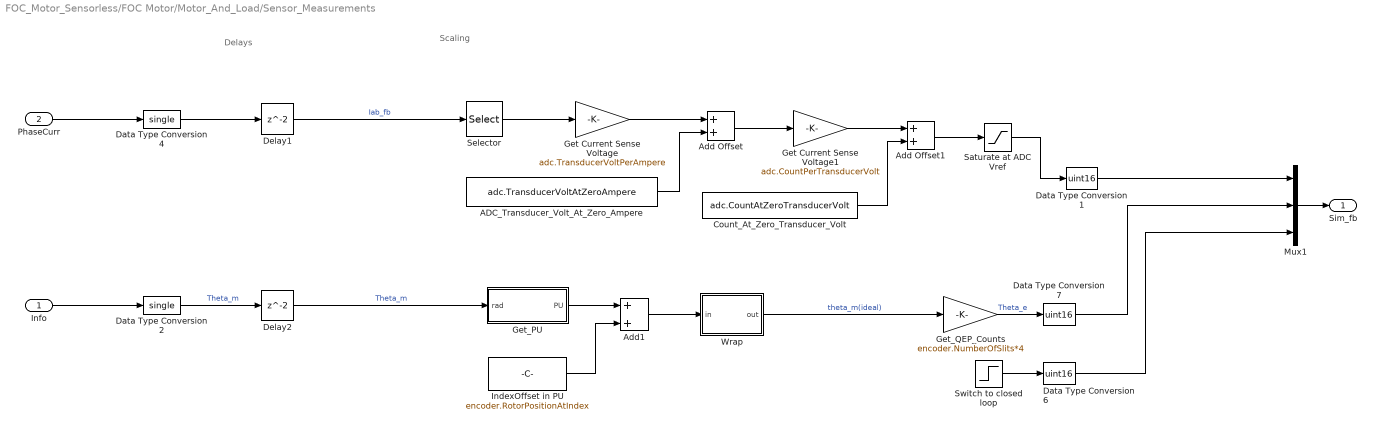
== system FOC_Motor_Sensorless/FOC Motor/Motor_And_Load/Sensor_Measurements ==
  note: Scaling
  note: Delays
  Info : Inport
  PhaseCurr : Inport  Port=2
  ADC_Transducer_Volt_At_Zero_Ampere : Constant  Value=adc.TransducerVoltAtZeroAmpere  OutDataTypeStr=single
  Add Offset : Sum  RndMeth=Simplest
  Add Offset1 : Sum  RndMeth=Simplest
  Add1 : Sum  RndMeth=Simplest
  Count_At_Zero_Transducer_Volt : Constant  Value=adc.CountAtZeroTransducerVolt  OutDataTypeStr=single  SampleTime=-1
  Data Type Conversion1 : DataTypeConversion  OutDataTypeStr=uint16  RndMeth=Simplest  SaturateOnIntegerOverflow=off
  Data Type Conversion2 : DataTypeConversion  OutDataTypeStr=single  RndMeth=Simplest  SaturateOnIntegerOverflow=off
  Data Type Conversion4 : DataTypeConversion  OutDataTypeStr=single  RndMeth=Simplest  SaturateOnIntegerOverflow=off
  Data Type Conversion6 : DataTypeConversion  OutDataTypeStr=uint16  RndMeth=Simplest  SaturateOnIntegerOverflow=off
  Data Type Conversion7 : DataTypeConversion  OutDataTypeStr=uint16  RndMeth=Simplest  SaturateOnIntegerOverflow=off
  Delay1 : Delay
  Delay2 : Delay
  Get Current Sense Voltage : Gain  Gain=adc.TransducerVoltPerAmpere  RndMeth=Simplest  OutDataTypeStr=Inherit: Same as input
  Get Current Sense Voltage1 : Gain  Gain=adc.CountPerTransducerVolt  RndMeth=Simplest  OutDataTypeStr=Inherit: Same as input
  "Get_PU " : Subsystem
  Get_QEP_Counts : Gain  Gain=encoder.NumberOfSlits*4  OutDataTypeStr=uint16  RndMeth=Simplest
  IndexOffset in PU : Constant  Value=encoder.RotorPositionAtIndex  OutDataTypeStr=single  SampleTime=-1
  Mux1 : Mux  Inputs=3
  Saturate at ADC Vref : Saturate  UpperLimit=adc.CountMax  LowerLimit=adc.CountMin
  Selector : Selector  InputPortWidth=3  IndexOptions=Index vector (dialog)  Indices=[1 2]  OutputSizes=1
  "Switch to closed loop " : Step  SampleTime=sampleTime.CurrentControl/2
  Wrap : Subsystem
  Sim_fb : Outport  VectorParamsAs1DForOutWhenUnconnected=off
  wires:
  Delay1/1 -> Selector/1  "Iab_fb"
  Data Type Conversion4/1 -> Delay1/1
  PhaseCurr/1 -> Data Type Conversion4/1
  Info/1 -> Data Type Conversion2/1
  Mux1/1 -> Sim_fb/1
  Data Type Conversion2/1 -> Delay2/1  "Theta_m"
  Add1/1 -> Wrap/1(in)
  Delay2/1 -> "Get_PU "/1(rad)  "Theta_m"
  Wrap/1(out) -> Get_QEP_Counts/1  "theta_m(ideal)"
  "Get_PU "/1(PU) -> Add1/1
  Get_QEP_Counts/1 -> Data Type Conversion7/1  "Theta_e"
  IndexOffset in PU/1 -> Add1/2
  "Switch to closed loop "/1 -> Data Type Conversion6/1
  Get Current Sense Voltage/1 -> Add Offset/1
  Saturate at ADC Vref/1 -> Data Type Conversion1/1
  Add Offset/1 -> Get Current Sense Voltage1/1
  Selector/1 -> Get Current Sense Voltage/1
  Data Type Conversion7/1 -> Mux1/2
  Data Type Conversion6/1 -> Mux1/3
  ADC_Transducer_Volt_At_Zero_Ampere/1 -> Add Offset/2
  Get Current Sense Voltage1/1 -> Add Offset1/1
  Add Offset1/1 -> Saturate at ADC Vref/1
  Count_At_Zero_Transducer_Volt/1 -> Add Offset1/2
  Data Type Conversion1/1 -> Mux1/1

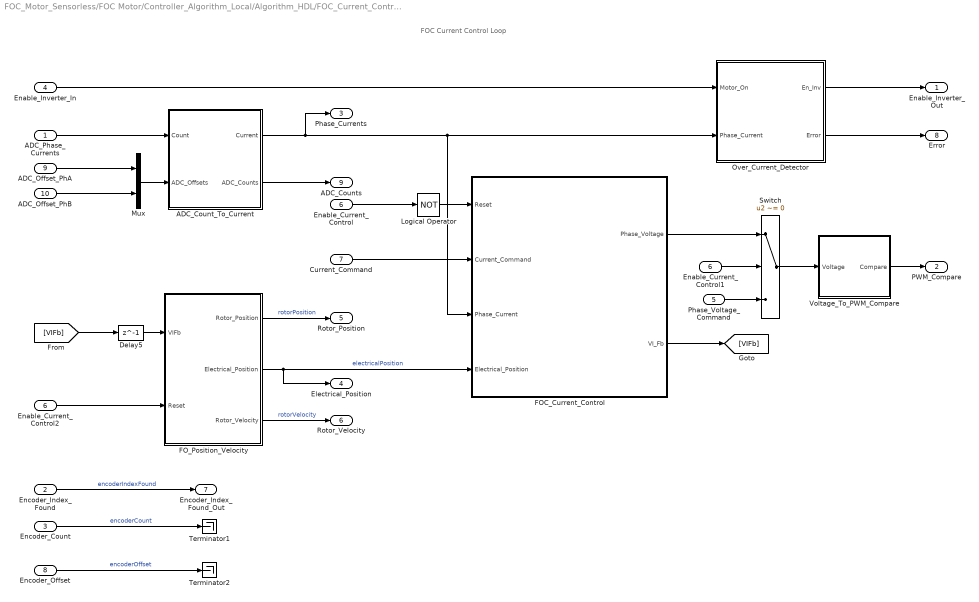
== system FOC_Motor_Sensorless/FOC Motor/Controller_Algorithm_Local/Algorithm_HDL/FOC_Current_Control ==
  note: FOC Current Control Loop
  ADC_Phase_Currents : Inport
  Encoder_Index_Found : Inport  Port=2  OutDataTypeStr=boolean  LockScale=on
  Encoder_Count : Inport  Port=3  OutDataTypeStr=uint16  LockScale=on
  Enable_Inverter_In : Inport  Port=4  OutDataTypeStr=boolean  LockScale=on
  Phase_Voltage_Command : Inport  Port=5
  Enable_Current_Control : Inport  Port=6  OutMin=0  OutMax=1  OutDataTypeStr=boolean
  Current_Command : Inport  Port=7
  Encoder_Offset : Inport  Port=8  OutDataTypeStr=fixdt(1,16,12)
  ADC_Offset_PhA : Inport  Port=9  OutDataTypeStr=uint16
  ADC_Offset_PhB : Inport  Port=10  OutDataTypeStr=uint16
  ADC_Count_To_Current : Subsystem
  Delay5 : Delay  DelayLength=1
  Enable_Current_Control1 : InportShadow  Port=6  OutMin=0  OutMax=1  OutDataTypeStr=boolean
  Enable_Current_Control2 : InportShadow  Port=6  OutMin=0  OutMax=1  OutDataTypeStr=boolean
  FOC_Current_Control : Subsystem  VariantControl=FixedPoint
  FO_Position_Velocity : Subsystem  VariantControl=ctrlVariantPosSns==PosSnsEnum.Encoder
  Logical Operator : Logic  Operator=NOT  IconShape=distinctive  AllPortsSameDT=off  OutDataTypeStr=boolean
  Mux : Mux  Inputs=2
  Over_Current_Detector : Subsystem
      mask Display: %fprintf('Detect\nOvercurrent')
  Switch : Switch  Criteria=u2 ~= 0  SaturateOnIntegerOverflow=off  InputSameDT=off
  Terminator1 : Terminator
  Terminator2 : Terminator
  Voltage_To_PWM_Compare : Subsystem
  Enable_Inverter_Out : Outport  OutMin=0  OutMax=1  VectorParamsAs1DForOutWhenUnconnected=off
  PWM_Compare : Outport  Port=2  VectorParamsAs1DForOutWhenUnconnected=off
  Phase_Currents : Outport  Port=3  VectorParamsAs1DForOutWhenUnconnected=off
  Electrical_Position : Outport  Port=4  VectorParamsAs1DForOutWhenUnconnected=off
  Rotor_Position : Outport  Port=5  VectorParamsAs1DForOutWhenUnconnected=off
  Rotor_Velocity : Outport  Port=6  VectorParamsAs1DForOutWhenUnconnected=off
  Encoder_Index_Found_Out : Outport  Port=7  OutMin=0  OutMax=1  VectorParamsAs1DForOutWhenUnconnected=off
  Error : Outport  Port=8  OutMin=0  OutMax=1  VectorParamsAs1DForOutWhenUnconnected=off
  ADC_Counts : Outport  Port=9  VectorParamsAs1DForOutWhenUnconnected=off
  wires:
  FO_Position_Velocity/2(Electrical_Position) -> FOC_Current_Control/4(Electrical_Position), Electrical_Position/1  "electricalPosition"
  Over_Current_Detector/2(Error) -> Error/1
  ADC_Phase_Currents/1 -> ADC_Count_To_Current/1(Count)
  Phase_Voltage_Command/1 -> Switch/3
  ADC_Count_To_Current/1(Current) -> Phase_Currents/1, FOC_Current_Control/3(Phase_Current), Over_Current_Detector/2(Phase_Current)
  FO_Position_Velocity/1(Rotor_Position) -> Rotor_Position/1  "rotorPosition"
  Voltage_To_PWM_Compare/1(Compare) -> PWM_Compare/1
  Switch/1 -> Voltage_To_PWM_Compare/1(Voltage)
  Enable_Current_Control/1 -> Logical Operator/1
  Enable_Current_Control1/1 -> Switch/2
  Enable_Inverter_In/1 -> Over_Current_Detector/1(Motor_On)
  Encoder_Index_Found/1 -> Encoder_Index_Found_Out/1  "encoderIndexFound"
  Over_Current_Detector/1(En_Inv) -> Enable_Inverter_Out/1
  Logical Operator/1 -> FOC_Current_Control/1(Reset)
  Current_Command/1 -> FOC_Current_Control/2(Current_Command)
  FOC_Current_Control/1(Phase_Voltage) -> Switch/1
  ADC_Offset_PhA/1 -> Mux/1
  ADC_Offset_PhB/1 -> Mux/2
  Mux/1 -> ADC_Count_To_Current/2(ADC_Offsets)
  ADC_Count_To_Current/2(ADC_Counts) -> ADC_Counts/1
  Delay5/1 -> FO_Position_Velocity/1(VIFb)
  Enable_Current_Control2/1 -> FO_Position_Velocity/2(Reset)
  FOC_Current_Control/2(VI_Fb) -> [VIFb]
  [VIFb] -> Delay5/1
  FO_Position_Velocity/3(Rotor_Velocity) -> Rotor_Velocity/1  "rotorVelocity"
  Encoder_Count/1 -> Terminator1/1  "encoderCount"
  Encoder_Offset/1 -> Terminator2/1  "encoderOffset"

== system FOC_Motor_Sensorless/FOC Motor/Controller_Algorithm_Local/Algotithm_C/ADC_Calibration ==
  note: ADC Calibration
  ADC_Counts_Ph_A : Inport
  ADC_Counts_Ph_B : Inport  Port=2
  Enable : EnablePort
      settings: AttributesFormatString=|
      | ----------------------------------------
      | States when enabling = %<StatesWhenEnabling>
  Constant : Constant  Value=paramAdcCalibrationSamples  OutDataTypeStr=single
  Constant1 : Constant  Value=paramAdcEnablecalibration  OutDataTypeStr=boolean
  Constant2 : Constant  Value=paramAdcCountAtZeroAmpere  OutDataTypeStr=single
  Data Type Conversion : DataTypeConversion  OutDataTypeStr=single  SaturateOnIntegerOverflow=off  RndMeth=Floor
  MATLAB Function : MATLAB Function  TreatAsAtomicUnit=on
  Mux : Mux  Inputs=2
  ADCOffsetPhA : Outport  InitialOutput=0  VectorParamsAs1DForOutWhenUnconnected=off
  ADCOffsetPhB : Outport  Port=2  InitialOutput=0  VectorParamsAs1DForOutWhenUnconnected=off
  ADCCaFlag : Outport  Port=3  InitialOutput=0  VectorParamsAs1DForOutWhenUnconnected=off
  wires:
  ADC_Counts_Ph_A/1 -> Mux/1
  ADC_Counts_Ph_B/1 -> Mux/2
  Mux/1 -> Data Type Conversion/1
  Constant/1 -> MATLAB Function/2(Samples)
  Constant1/1 -> MATLAB Function/3(EnCalibration)
  Data Type Conversion/1 -> MATLAB Function/1(ADCCounts)
  Constant2/1 -> MATLAB Function/4(ADCOffsets)
  MATLAB Function/3(Flag) -> ADCCaFlag/1
  MATLAB Function/2(ADCOffsetPhB) -> ADCOffsetPhB/1
  MATLAB Function/1(ADCOffsetPhA) -> ADCOffsetPhA/1

== system FOC_Motor_Sensorless/FOC Motor/Controller_Algorithm_Local/Algotithm_C/Open_Loop_Velocity_Control ==
  note: Open_Loop_Velocity_Control
  note: Open Loop Velocity Control
  note: Open Loop Velocity Control
  Velocity_Command : Inport
  Enable : EnablePort  StatesWhenEnabling=reset
      settings: AttributesFormatString=|
      | ----------------------------------------
      | States when enabling = %<StatesWhenEnabling>
  Constant : Constant  Value=0.1  OutDataTypeStr=single
  Constant1 : Constant  Value=0.1*inverter.V_dc/sqrt(3)  OutDataTypeStr=single
  Constant2 : Constant  Value=0  OutDataTypeStr=single
  Inverse Park Transform : mcbeeMathTransformLib/Park to Clarke Angle Transform  AxisAlignment=D-axis  UseWithEmbedded=on  PhaseInput=Two inputs  ThetaInput=Sine and Cosine electrical position  AngleInput=Per-unit  N_points=1024
      settings: LibrarySourceBlock=mcbcontrolslib/Inverse Park Transform
  Mux : Mux  Inputs=3
  Open_Loop_Control : Subsystem
  PWM Reference Generator : mcbcontrolslib/PWM Reference Generator  inSignal=Valphabeta  modType=SVM: space vector modulation
      settings: LibrarySourceBlock=mcblib/Controls/Math Transforms/PWM Reference Generator
  Product : Product  OutDataTypeStr=single
  Sign : Signum
  Sine-Cosine Lookup : mcbcontrolslib/SinCos Embedded Optimized  LabelModeActiveChoice=MCB_Sin  OptforProc=off  ApproximationMethod=None  UserApproxMethod=Lookup  ApproxStatus=None  InterpMethod=Linear point-slope  NumberOfDataPoints=16  NumberOfIterations=11  RemoveProtectionAgainstOutOfRangeInput=off  TableDataTypeStr=Inherit: Inherit via input  AngleInput=Per-unit  ThetaDataType=single  N_points=1024  DatatypeInput=Inherit from input  Datatype=Inherit: Same as input
  Phase_Voltage : Outport  VectorParamsAs1DForOutWhenUnconnected=off
  wires:
  Mux/1 -> Phase_Voltage/1  "phaseVoltage"
  Inverse Park Transform/2 -> PWM Reference Generator/2
  Inverse Park Transform/1 -> PWM Reference Generator/1
  PWM Reference Generator/3 -> Mux/3
  PWM Reference Generator/2 -> Mux/2
  PWM Reference Generator/1 -> Mux/1
  Sine-Cosine Lookup/2 -> Inverse Park Transform/4
  Sine-Cosine Lookup/1 -> Inverse Park Transform/3
  Open_Loop_Control/1(Pos_PU_Out) -> Sine-Cosine Lookup/1
  Product/1 -> Open_Loop_Control/1(OpenLoopSpeed)
  Constant/1 -> Product/2
  Sign/1 -> Product/1
  Velocity_Command/1 -> Sign/1
  Constant2/1 -> Inverse Park Transform/2
  Constant1/1 -> Inverse Park Transform/1

== system FOC_Motor_Sensorless/FOC Motor/Controller_Algorithm_Local/Algotithm_C/StandBy ==
  note: Disabled
  Enable : EnablePort
      settings: AttributesFormatString=|
      | ----------------------------------------
      | States when enabling = %<StatesWhenEnabling>
  Constant : Constant  Value=[0 0 0]  OutDataTypeStr=Inherit: Inherit via back propagation
  Phase Voltage : Outport  InitialOutput=[0 0 0]  VectorParamsAs1DForOutWhenUnconnected=off
      settings: AttributesFormatString=--------------------------------------------\nInitial Output = %<InitialOutput>
  wires:
  Constant/1 -> Phase Voltage/1

== system FOC_Motor_Sensorless/FOC Motor/Controller_Algorithm_Local/Algotithm_C/Velocity_Control ==
  note: Velocity Control
  Velocity_Command : Inport
  Velocity_Measured : Inport  Port=2
  Enable : EnablePort  StatesWhenEnabling=reset
      settings: AttributesFormatString=|
      | ----------------------------------------
      | States when enabling = %<StatesWhenEnabling>
  Velocity_Control : Subsystem
  Q_Current_Command : Outport  InitialOutput=0  VectorParamsAs1DForOutWhenUnconnected=off
  wires:
  Velocity_Command/1 -> Velocity_Control/1(Velocity_Command)
  Velocity_Measured/1 -> Velocity_Control/2(Velocity_Measured)  "rotorVelocity"
  Velocity_Control/1(Current) -> Q_Current_Command/1  "qCurrentCommand"

== system FOC_Motor_Sensorless/FOC Motor/Motor_And_Load/Plant /MCB ==
  Vabc : Inport
  InverterEnable : Inport  Port=2
  Load : Inport  Port=3
  Bus Selector : BusSelector  OutputSignals=MtrPos
  Inverter : Subsystem
  PWM_Count_to_Duty : Subsystem
  Surface Mount PMSM : autolibpmsmexterior/Surface Mount PMSM  port_config=Torque  sim_type=Discrete  Ts=sampleTime.CurrentControl/2  P=pmsm.p  Rs=pmsm.Rs  Ldq_=pmsm.Ld  KConstText=Permanent flux linkage constant (lambda_pm):  lambda_pm=pmsm.FluxPM  Ke=159.9771  Kt=1.323  mechanical=[pmsm.J, pmsm.B, 0]  idq0=[0 0]  theta_init=0  omega_init=0  KConst=pmsm.FluxPM  lambda_pm_calc=pmsm.FluxPM  RefBlkName='autolibpmsmexterior/Surface Mount PMSM'  aMode=5  Ldq="[0.0002      0.0002]"
  Terminator : Terminator
  Theta : Outport
  Iabc : Outport  Port=2
  MotorSpeed : Outport  Port=3
  wires:
  Surface Mount PMSM/2 -> Iabc/1  "Iabc_motor"
  Load/1 -> Surface Mount PMSM/1
  Surface Mount PMSM/1 -> Bus Selector/1
  Bus Selector/1 -> Theta/1  "<MtrPos>"
  Vabc/1 -> PWM_Count_to_Duty/1(<pwmCompare>)
  InverterEnable/1 -> Terminator/1
  Surface Mount PMSM/3 -> MotorSpeed/1  "motorspeed"
  PWM_Count_to_Duty/1(Duty) -> Inverter/1(Duty)
  Inverter/1(Vabc_motor) -> Surface Mount PMSM/2
